simulink model "motor"  (R2020b)
settings: Solver=VariableStepAuto  StartTime=0.0  StopTime=0.4  RelTol=1e-3
model workspace (MAT data in the model file):
  J = Simulink.Parameter
  J.Value = 3.2284e-06
  J.DataType = 'auto'
  J.Dimensions = [1 1]
  Kd = Simulink.Parameter
  Kd.Value = 0.48976
  Kd.DataType = 'auto'
  Kd.Dimensions = [1 1]
  Ke = Simulink.Parameter
  Ke.Value = 0.0274
  Ke.DataType = 'auto'
  Ke.Dimensions = [1 1]
  Ki = Simulink.Parameter
  Ki.Value = 4810.143
  Ki.DataType = 'auto'
  Ki.Dimensions = [1 1]
  Kp = Simulink.Parameter
  Kp.Value = 97.11
  Kp.DataType = 'auto'
  Kp.Dimensions = [1 1]
  Kt = Simulink.Parameter
  Kt.Value = 0.0274
  Kt.DataType = 'auto'
  Kt.Dimensions = [1 1]
  L = Simulink.Parameter
  L.Value = 2.75e-06
  L.DataType = 'auto'
  L.Dimensions = [1 1]
  N = Simulink.Parameter
  N.Value = 100000
  N.DataType = 'auto'
  N.Dimensions = [1 1]
  R = Simulink.Parameter
  R.Value = 4
  R.DataType = 'auto'
  R.Dimensions = [1 1]
  b = Simulink.Parameter
  b.Value = 3.5077e-06
  b.DataType = 'auto'
  b.Dimensions = [1 1]
settings Model: DataDictionary=motor.sldd  OrderedModelArguments=off  Creator=sushma  LastModifiedBy=sushma

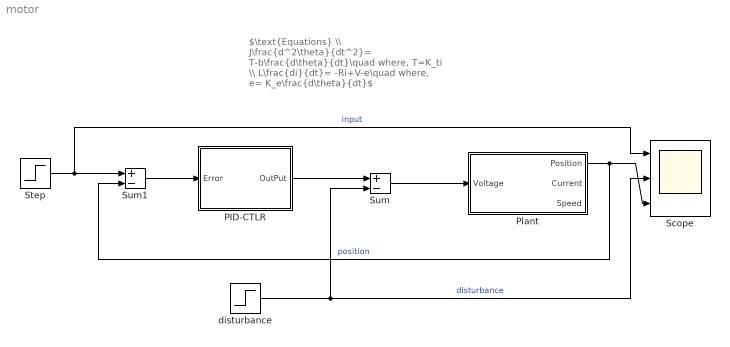
== system motor ==
  note: $\text{Equations} \\ J\frac{d^2\theta}{dt^2}= T-b\frac{d\theta}{dt}\quad where, T=K_ti \\ L\frac{di}{dt}= -Ri+V-e\quad where, e= K_e\frac{d\theta}{dt}$
  PID-CTLR : Subsystem
  Plant : Subsystem
  Scope : Scope  NumInputPorts=3
  Step : Step  Time=0.2  SampleTime=0
  Sum : Sum  Inputs=+-
  Sum1 : Sum  Inputs=+-
  disturbance : Step  SampleTime=0
  wires:
  PID-CTLR/1(OutPut) -> Sum/1
  Sum1/1 -> PID-CTLR/1(Error)
  Sum/1 -> Plant/1(Voltage)
  Plant/1(Position) -> Sum1/2, Scope/3  "position"
  Step/1 -> Scope/1, Sum1/1  "input"
  disturbance/1 -> Scope/2, Sum/2  "disturbance"

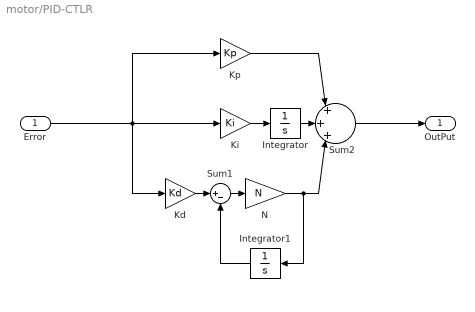
== system motor/PID-CTLR ==
  Error : Inport  OutDataTypeStr=double  PortDimensions=1  SampleTime=0
  Integrator : Integrator
  Integrator1 : Integrator
  Kd : Gain  Gain=Kd
  Ki : Gain  Gain=Ki
  Kp : Gain  Gain=Kp
  N : Gain  Gain=N
  Sum1 : Sum  Inputs=|+-
  Sum2 : Sum  Inputs=|+|+|+|
  OutPut : Outport  OutDataTypeStr=double  PortDimensions=1  SampleTime=0
  wires:
  Ki/1 -> Integrator/1
  Sum2/1 -> OutPut/1
  N/1 -> Sum2/3, Integrator1/1
  Integrator1/1 -> Sum1/2
  Integrator/1 -> Sum2/2
  Kp/1 -> Sum2/1
  Error/1 -> Kd/1, Kp/1, Ki/1
  Kd/1 -> Sum1/1
  Sum1/1 -> N/1

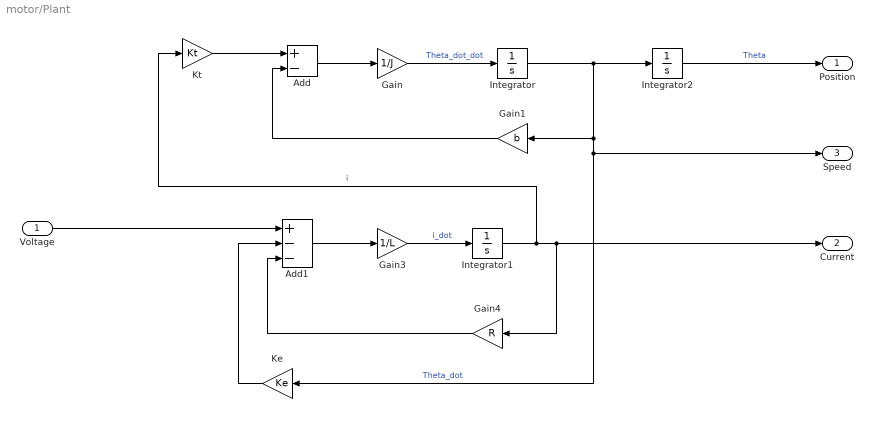
== system motor/Plant ==
  Voltage : Inport
  Add : Sum  Inputs=+-
  Add1 : Sum  Inputs=+--
  Gain : Gain  Gain=1/J
  Gain1 : Gain  Gain=b
  Gain3 : Gain  Gain=1/L
  Gain4 : Gain  Gain=R
  Integrator : Integrator
  Integrator1 : Integrator
  Integrator2 : Integrator
  Ke : Gain  Gain=Ke
  Kt : Gain  Gain=Kt
  Position : Outport
  Current : Outport  Port=2
  Speed : Outport  Port=3
  wires:
  Kt/1 -> Add/1
  Gain3/1 -> Integrator1/1  "i_dot"
  Voltage/1 -> Add1/1
  Gain/1 -> Integrator/1  "Theta_dot_dot"
  Add1/1 -> Gain3/1
  Integrator1/1 -> Kt/1, Current/1, Gain4/1  "i"
  Add/1 -> Gain/1
  Ke/1 -> Add1/2
  Integrator/1 -> Integrator2/1, Speed/1, Ke/1, Gain1/1  "Theta_dot"
  Gain4/1 -> Add1/3
  Integrator2/1 -> Position/1  "Theta"
  Gain1/1 -> Add/2
